simulink model "GatewayMavlinkProtocol"  (R2025b)
settings: Solver=FixedStepDiscrete  StartTime=0.0  StopTime=inf  FixedStep=0.01  RelTol=1e-3
model workspace (MAT data in the model file):
  UDPMessageLength = 10
undefined symbols (not defined in the file): f
libraries: uavmavlinklib x9, instrumentlib x4
settings Model: Creator=The MathWorks, Inc.  LastModifiedBy=89447
settings OptimizationCC: DefaultParameterBehavior=Inlined  EnhancedBackFolding=on  PassReuseOutputArgsAs=Individual arguments  ZeroExternalMemoryAtStartup=off  ZeroInternalMemoryAtStartup=off  MaxStackSize=64  OptimizeBlockOrder=speed  DifferentSizesBufferReuse=on  OptimizationCustomize=off  EfficientTunableParamExpr=on
settings HardwareCC: TargetBitPerLong=64.0  TargetBitPerPointer=64.0  TargetBitPerSizeT=64.0  TargetBitPerPtrDiffT=64.0  TargetLargestAtomicFloat=Float  TargetIntDivRoundTo=Zero  TargetEndianess=LittleEndian  TargetWordSize=64.0  TargetHWDeviceType=Intel->x86-64 (Linux 64)  ProdEqTarget=off
settings ModelReferenceCC: ModelReferenceNumInstancesAllowed=Single  SupportModelReferenceSimTargetCustomCode=on
settings SFSimCC: SimUserSources=D:\MATLAB\R2025b\toolbox\eml\externalDependency\timefun\coder_posix_time.c  SimUserIncludeDirs=D:\MATLAB\R2025b\toolbox\eml\externalDependency\timefun
settings RTWCC: SystemTargetFile=ert.tlc  GenCodeOnly=on  TemplateMakefile=ert_default_tmf  CustomInclude=D:\MATLAB\R2025b\toolbox\eml\externalDependency\timefun  CustomSource=D:\MATLAB\R2025b\toolbox\eml\externalDependency\timefun\coder_posix_time.c  TargetLang=C++  Description=Embedded Coder
settings CodeAppCC: ForceParamTrailComments=on  IgnoreCustomStorageClasses=off  OperatorAnnotations=on  SimulinkDataObjDesc=on  SFDataObjDesc=on  InsertBlockDesc=on
settings ERTTargetCC: ExtModeTransport=2.0  ExtModeStaticAlloc=on  ExtModeMexFile=ext_xcp  ExtModeIntrfLevel=Level2 - Open  ERTCustomFileTemplate=example_file_process.tlc  TargetLangStandard=C++11 (ISO)  SubcomponentCodeInterfacePackaging=Nonreusable function  SupportContinuousTime=on

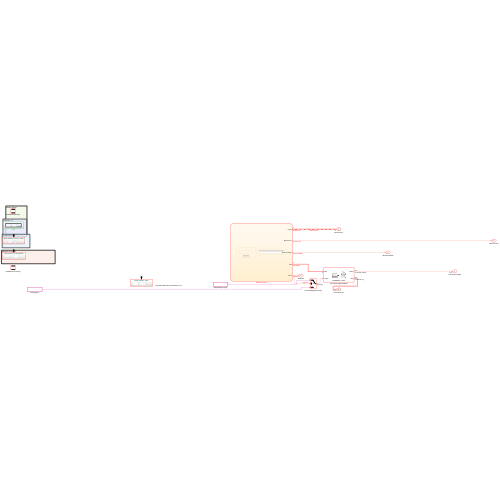
[thumbnail: Simulink's stored preview of the top-level diagram]
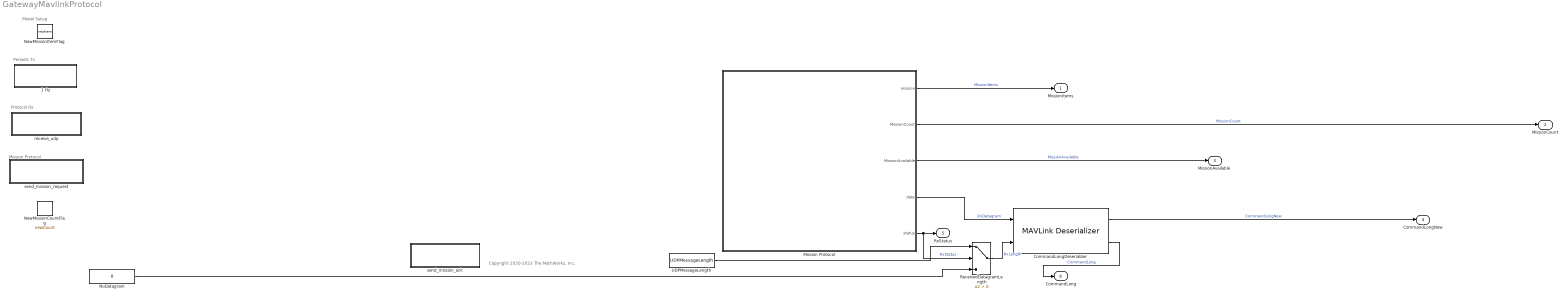
== system GatewayMavlinkProtocol ==
  note: Periodic Tx
  note: Model Setup
  note: Protocol Rx
  note: Mission Protocol
  note: Copyright 2020-2023 The MathWorks, Inc.
  1 Hz : Subsystem
  CommandLongDeserializer : uavmavlinklib/MAVLink Deserializer  dialectSource=Select from standard MAVLink dialects  dialect=common.xml  dialectCustom=common.xml  version=2  messageType=COMMAND_LONG  inputDataLength=on  SystemIDFilter=off  systemID=1  ComponentIDFilter=off  componentID=1  queueMsg=off  queueMsgSize=50  dropNum=off
  Mission Protocol : Stateflow chart  TreatAsAtomicUnit=on  SystemSampleTime=0.01
  NewMissionCountFlag : DataStoreMemory  DataStoreName=newCount  InitialValue=boolean(0)  ShowAdditionalParam=off  OutDataTypeStr=boolean
  NewMissionItemFlag : DataStoreMemory  DataStoreName=newItem  InitialValue=boolean(0)  ShowAdditionalParam=off  OutDataTypeStr=boolean
  NoDatagram : Constant  Value=0
  ReceivedDatagramLength : Switch  Criteria=u2 > Threshold
  UDPMessageLength : Constant  Value=UDPMessageLength
  receive_udp : Subsystem  TreatAsAtomicUnit=on
  send_mission_ack : Subsystem  TreatAsAtomicUnit=on
  send_mission_request : Subsystem  TreatAsAtomicUnit=on
  MissionItems : Outport  OutDataTypeStr=Bus: SL_Bus_MAVLink_MISSION_ITEM_INT_Payload  BusOutputAsStruct=on
  MissionCount : Outport  Port=2
  MissionAvailable : Outport  Port=3
  CommandLongNew : Outport  Port=4
  RxStatus : Outport  Port=5
  CommandLong : Outport  Port=6  OutDataTypeStr=Bus: SL_Bus_MAVLink_COMMAND_LONG_Packet
  wires:
  Mission Protocol/1(mission) -> MissionItems/1  "MissionItems"
  Mission Protocol/2(MissionCount) -> MissionCount/1  "MissionCount"
  Mission Protocol/3(MissionAvailable) -> MissionAvailable/1  "MissionAvailable"
  Mission Protocol/4(data) -> CommandLongDeserializer/1  "RxDatagram"
  Mission Protocol/5(status) -> ReceivedDatagramLength/2, RxStatus/1  "RxStatus"
  UDPMessageLength/1 -> ReceivedDatagramLength/1
  NoDatagram/1 -> ReceivedDatagramLength/3
  CommandLongDeserializer/1 -> CommandLongNew/1  "CommandLongNew"
  CommandLongDeserializer/2 -> CommandLong/1  "CommandLong"
  ReceivedDatagramLength/1 -> CommandLongDeserializer/2  "RxLength"

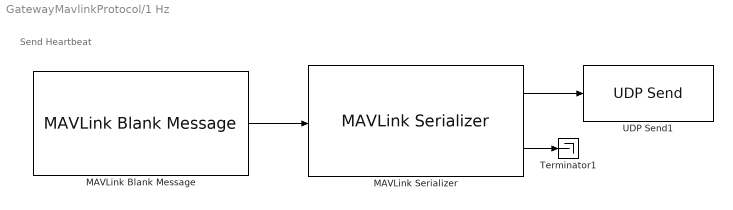
== system GatewayMavlinkProtocol/1 Hz ==
  note: Send Heartbeat
  MAVLink Blank Message : uavmavlinklib/MAVLink Blank Message  dialectSource=Select from standard MAVLink dialects  dialect=common.xml  dialectCustom=D:\Sandbox\Buav\matlab\toolbox\uav\uavmatlab\mavlink\message_definitions\ardupilotmega.xml  version=2  messageType=HEARTBEAT  SystemID=1  ComponentID=1  SampleTime=1
  MAVLink Serializer : uavmavlinklib/MAVLink Serializer  dialectSource=Select from standard MAVLink dialects  dialect=common.xml  dialectCustom=common.xml  version=2  messageType=HEARTBEAT
  Terminator1 : Terminator
  UDP Send1 : instrumentlib/UDP Send  Host=127.0.0.1  Port=14550  LocalAddress=localhost  LocalPort=-1  EnablePortSharing=on  OutputDatagramPacketSize=512  ByteOrder=big-endian  EnableBlockingMode=off  SimulateUsing=Interpreted execution
  wires:
  MAVLink Serializer/2 -> Terminator1/1
  MAVLink Blank Message/1 -> MAVLink Serializer/1
  MAVLink Serializer/1 -> UDP Send1/1

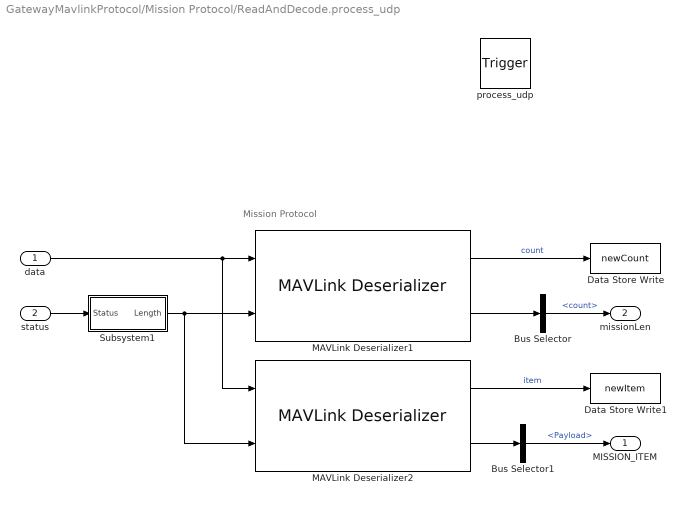
== system GatewayMavlinkProtocol/Mission Protocol/ReadAndDecode.process_udp ==
  note: Mission Protocol
  data : Inport  OutDataTypeStr=uint8  PortDimensions=UDPMessageLength
  status : Inport  Port=2  OutDataTypeStr=double  PortDimensions=1
  process_udp : TriggerPort  TriggerType=function-call  VariantControl=(inherit)
      settings: CopyFcn=Stateflow.SLINSF.SimulinkMan.removeBlockPreDeleteFcn  PreDeleteFcn=Stateflow.SLINSF.SimulinkMan.unsafePredeleteFcn
  Bus Selector : BusSelector  OutputSignals=Payload.count
  Bus Selector1 : BusSelector  OutputSignals=Payload
  Data Store Write : DataStoreWrite  DataStoreName=newCount  IndexOptions=Index vector (dialog)  Indices=1  OutputSizes=1
  Data Store Write1 : DataStoreWrite  DataStoreName=newItem  IndexOptions=Index vector (dialog)  Indices=1  OutputSizes=1
  MAVLink Deserializer1 : uavmavlinklib/MAVLink Deserializer  dialectSource=Select from standard MAVLink dialects  dialect=common.xml  dialectCustom=common.xml  version=2  messageType=MISSION_COUNT  inputDataLength=on  SystemIDFilter=off  systemID=1  ComponentIDFilter=off  componentID=1  queueMsg=off  queueMsgSize=50  dropNum=off
  MAVLink Deserializer2 : uavmavlinklib/MAVLink Deserializer  dialectSource=Select from standard MAVLink dialects  dialect=common.xml  dialectCustom=common.xml  version=2  messageType=MISSION_ITEM_INT  inputDataLength=on  SystemIDFilter=off  systemID=1  ComponentIDFilter=off  componentID=1  queueMsg=off  queueMsgSize=50  dropNum=off
  Subsystem1 : Subsystem
  MISSION_ITEM : Outport
  missionLen : Outport  Port=2
  wires:
  data/1 -> MAVLink Deserializer1/1, MAVLink Deserializer2/1
  MAVLink Deserializer1/1 -> Data Store Write/1  "count"
  MAVLink Deserializer1/2 -> Bus Selector/1
  Bus Selector/1 -> missionLen/1  "<count>"
  MAVLink Deserializer2/1 -> Data Store Write1/1  "item"
  MAVLink Deserializer2/2 -> Bus Selector1/1
  Bus Selector1/1 -> MISSION_ITEM/1  "<Payload>"
  status/1 -> Subsystem1/1(Status)
  Subsystem1/1(Length) -> MAVLink Deserializer1/2, MAVLink Deserializer2/2

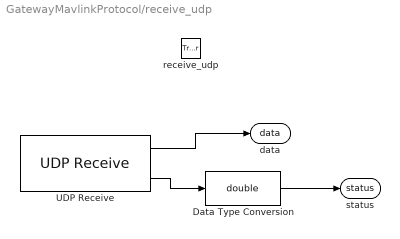
== system GatewayMavlinkProtocol/receive_udp ==
  receive_udp : TriggerPort  TriggerType=function-call  IsSimulinkFunction=on  FunctionName=receive_udp  FunctionVisibility=scoped  VariantControl=(inherit)
  Data Type Conversion : DataTypeConversion  OutDataTypeStr=double  SaturateOnIntegerOverflow=off  RndMeth=Floor
  UDP Receive : instrumentlib/UDP Receive  LocalAddress=localhost  LocalPort=-1  EnablePortSharing=on  Host=127.0.0.1  Port=14550  GetLatestData=off  DataSize=10  DataType=uint8  ASCIIFormatting=%f,  Terminator=LF  CustomTerminator=10  ByteOrder=big-endian  EnableBlockingMode=off  Timeout=10  SampleTime=-1  SimulateUsing=Interpreted execution
  data : ArgOut  DisableCoverage=on  OutDataTypeStr=uint8  PortDimensions=10  ArgumentName=data
  status : ArgOut  Port=2  ArgumentName=status
  wires:
  Data Type Conversion/1 -> status/1
  UDP Receive/1 -> data/1
  UDP Receive/2 -> Data Type Conversion/1

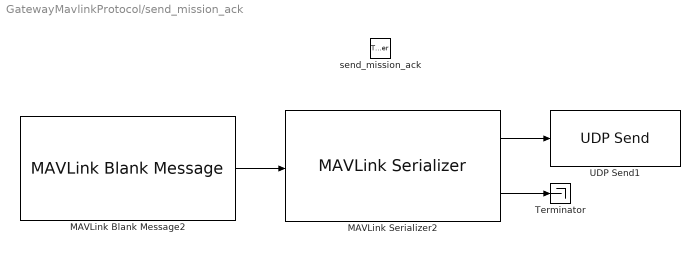
== system GatewayMavlinkProtocol/send_mission_ack ==
  send_mission_ack : TriggerPort  TriggerType=function-call  IsSimulinkFunction=on  FunctionName=send_mission_ack  FunctionVisibility=scoped  VariantControl=(inherit)
  MAVLink Blank Message2 : uavmavlinklib/MAVLink Blank Message  dialectSource=Select from standard MAVLink dialects  dialect=common.xml  dialectCustom=D:\Sandbox\Buav\matlab\toolbox\uav\uavmatlab\mavlink\message_definitions\ardupilotmega.xml  version=2  messageType=MISSION_ACK  SystemID=1  ComponentID=1  SampleTime=-1
  MAVLink Serializer2 : uavmavlinklib/MAVLink Serializer  dialectSource=Select from standard MAVLink dialects  dialect=common.xml  dialectCustom=common.xml  version=2  messageType=MISSION_ACK
  Terminator : Terminator
  UDP Send1 : instrumentlib/UDP Send  Host=127.0.0.1  Port=14550  LocalAddress=localhost  LocalPort=-1  EnablePortSharing=on  OutputDatagramPacketSize=512  ByteOrder=big-endian  EnableBlockingMode=off  SimulateUsing=Interpreted execution
  wires:
  MAVLink Blank Message2/1 -> MAVLink Serializer2/1
  MAVLink Serializer2/2 -> Terminator/1
  MAVLink Serializer2/1 -> UDP Send1/1

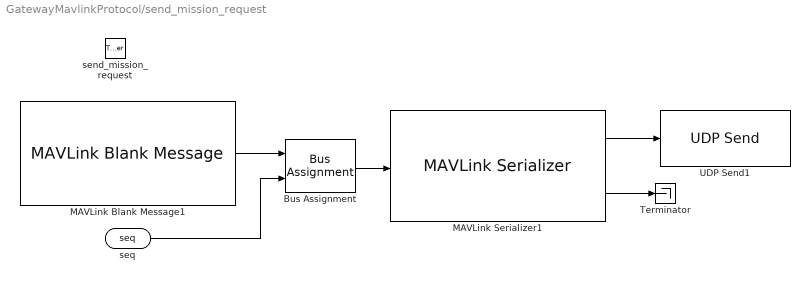
== system GatewayMavlinkProtocol/send_mission_request ==
  send_mission_request : TriggerPort  TriggerType=function-call  IsSimulinkFunction=on  FunctionName=send_mission_request  FunctionVisibility=scoped  VariantControl=(inherit)
  Bus Assignment : BusAssignment  AssignedSignals=Payload.seq
  MAVLink Blank Message1 : uavmavlinklib/MAVLink Blank Message  dialectSource=Select from standard MAVLink dialects  dialect=common.xml  dialectCustom=D:\Sandbox\Buav\matlab\toolbox\uav\uavmatlab\mavlink\message_definitions\ardupilotmega.xml  version=2  messageType=MISSION_REQUEST_INT  SystemID=1  ComponentID=1  SampleTime=-1
  MAVLink Serializer1 : uavmavlinklib/MAVLink Serializer  dialectSource=Select from standard MAVLink dialects  dialect=common.xml  dialectCustom=common.xml  version=2  messageType=MISSION_REQUEST_INT
  Terminator : Terminator
  UDP Send1 : instrumentlib/UDP Send  Host=127.0.0.1  Port=14550  LocalAddress=localhost  LocalPort=-1  EnablePortSharing=on  OutputDatagramPacketSize=512  ByteOrder=big-endian  EnableBlockingMode=off  SimulateUsing=Interpreted execution
  seq : ArgIn  OutDataTypeStr=uint16  ArgumentName=seq
  wires:
  MAVLink Serializer1/2 -> Terminator/1
  MAVLink Blank Message1/1 -> Bus Assignment/1
  Bus Assignment/1 -> MAVLink Serializer1/1
  seq/1 -> Bus Assignment/2
  MAVLink Serializer1/1 -> UDP Send1/1

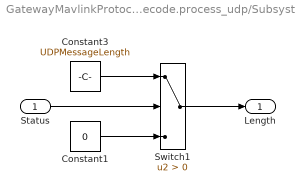
== system GatewayMavlinkProtocol/Mission Protocol/ReadAndDecode.process_udp/Subsystem1 ==
  Status : Inport
  Constant1 : Constant  Value=0
  Constant3 : Constant  Value=UDPMessageLength
  Switch1 : Switch  Criteria=u2 > Threshold  SaturateOnIntegerOverflow=off  InputSameDT=off
  Length : Outport
  wires:
  Status/1 -> Switch1/2
  Constant1/1 -> Switch1/3
  Constant3/1 -> Switch1/1
  Switch1/1 -> Length/1

== stateflow chart GatewayMavlinkProtocol/Mission Protocol ==
  state Process [parallel]
    settings: executionOrder=2
    state idle
    state receivingMission
      state sendRequest
        send_mission_request(currentWP)
      state waitForMissionItem
      state sendAck
        send_mission_ack;
      (default) -> sendRequest : {currentWP = uint16(0);
          | totalWPs = missionLen - uint16(1);
          | MissionCount = missionLen;
          | MissionAvailable = false;}
      waitForMissionItem -> sendRequest [order 1] : [(newItem == 1) && (currentWP < totalWPs ) ]
          | {currentWP = currentWP + uint16(1);
          | mission(currentWP) = MISSION_ITEM;}
      sendRequest -> waitForMissionItem
      waitForMissionItem -> sendAck [order 2] : [(newItem == 1) && (currentWP >= totalWPs )]
          | {currentWP = currentWP + uint16(1);
          | mission(currentWP) = MISSION_ITEM;
          | MissionCount = missionLen;
          | MissionAvailable = true;}
    (default) -> idle
    receivingMission -> idle : [MissionAvailable]
    idle -> receivingMission : [newCount == 1]
  state ReadAndDecode [parallel]
    [data, status] = receive_udp();
    [MISSION_ITEM, missionLen] = process_udp(data, status);
    settings: executionOrder=1
    state [MISSION_ITEM,missionLen] = process_udp(data,status) [function]
  data: data function_input uint8 size=UDPMessageLength; status function_input double size=1; MISSION_ITEM function_output; missionLen function_output; totalWPs local uint16; currentWP local uint16; mission output Bus: SL_Bus_MAVLink_MISSION_ITEM_INT_Payload size=10; MISSION_ITEM local Bus: SL_Bus_MAVLink_MISSION_ITEM_INT_Payload; missionLen local uint16 size=1 =uint16(0); newCount data_store_memory size=1 =boolean(0); newItem data_store_memory size=1 =boolean(0); MissionCount output uint16 size=1 =uint16(0); MissionAvailable output boolean size=1 =false; data output uint8 size=UDPMessageLength =uint8(zeros(UDPMessageLength,1)); status output double size=1 =0
